simulink model "PID666"  (R2024b)
settings: Solver=FixedStepDiscrete  StartTime=0.0  StopTime=inf  FixedStep=0.0001  RelTol=1e-3
undefined symbols (not defined in the file or in its folder): C28x, CPU1, CPU2, dspblkCoreblockFVToolHelper, gcbh
libraries: c2837xDlib x5, c280xlib x2, c2802xlib x1
settings Model: SimulationMode=external  ExtModeTrigDuration=8  Creator=lenovo  LastModifiedBy=chaiy
settings OptimizationCC: DefaultUnderspecifiedDataType=single  EnhancedBackFolding=on  PassReuseOutputArgsAs=Individual arguments  MaxStackSize=1024  OptimizeBlockOrder=speed  DifferentSizesBufferReuse=on  OptimizationCustomize=off  DenormalBehavior=FlushToZero  EfficientTunableParamExpr=on
settings DebuggingCC: ParameterTunabilityLossMsg=error
settings HardwareCC: ProdBitPerChar=16  ProdBitPerInt=16  ProdBitPerPointer=32  ProdBitPerSizeT=32  ProdBitPerPtrDiffT=32  ProdLargestAtomicInteger=Integer  ProdLargestAtomicFloat=None  ProdWordSize=16  ProdLongLongMode=on  ProdHWDeviceType=Texas Instruments->C2000
settings ModelReferenceCC: EnableRefExpFcnMdlSchedulingChecks=on  ModelReferenceNumInstancesAllowed=Single
settings SFSimCC: MATLABDynamicMemAlloc=off
settings RTWCC: Description=Embedded Coder  SystemTargetFile=ert.tlc  HardwareBoard=TI Delfino F28379D LaunchPad  TemplateMakefile=ert_default_tmf  Toolchain=Texas Instruments Code Composer Studio (C2000)  CodeProfilingSaveOptions=AllData  GPUComputeCapability=3.5
settings CodeAppCC: ForceParamTrailComments=on  IgnoreCustomStorageClasses=off  MaxIdLength=95  OperatorAnnotations=on  SimulinkDataObjDesc=on  SFDataObjDesc=on  InsertBlockDesc=on
settings ERTTargetCC: CodeReplacementLibrary=TI C28x  SupportContinuousTime=on  ExtMode=on  ExtModeTransport=4  ExtModeStaticAlloc=on  ExtModeMexFile=ext_xcp  ExtModeIntrfLevel=Level2 - Open  InlinedParameterPlacement=Hierarchical  DynamicArrayContainerType=coder::array

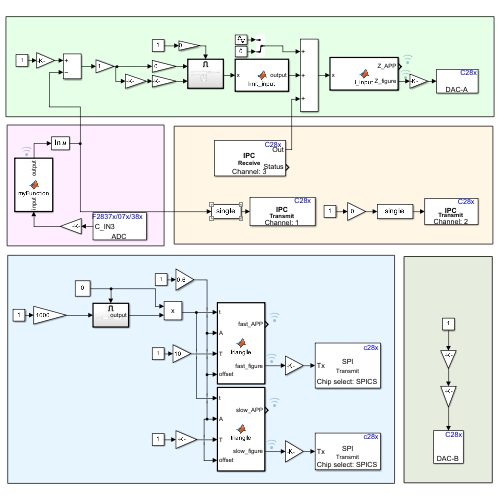
[thumbnail: Simulink's stored preview of the top-level diagram]
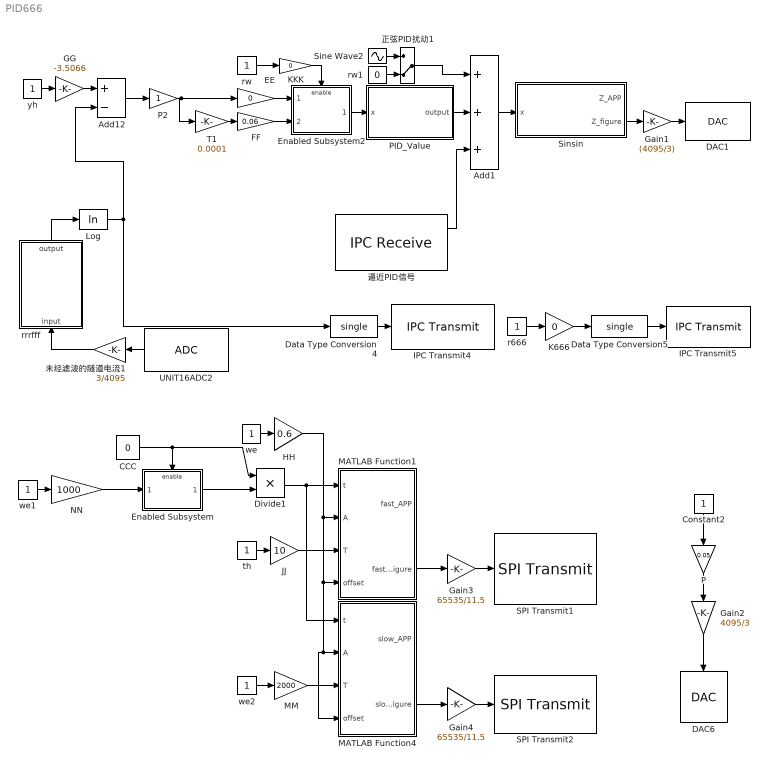
== system PID666 ==
  Add1 : Sum  Inputs=+++
  Add12 : Sum  Inputs=+-
  CCC : Constant  Value=0  SampleTime=0.0001
  Constant2 : Constant  SampleTime=0.0001
  DAC1 : c2837xDlib/DAC  channel=A  saturate=off
  DAC6 : c2837xDlib/DAC  channel=B  saturate=off
  Data Type Conversion4 : DataTypeConversion  OutDataTypeStr=single  SaturateOnIntegerOverflow=off  RndMeth=Floor
  Data Type Conversion5 : DataTypeConversion  OutDataTypeStr=single  SaturateOnIntegerOverflow=off  RndMeth=Floor
  Divide1 : Product  Inputs=**
  EE : Gain  Gain=0
  Enabled Subsystem : Subsystem  TreatAsAtomicUnit=on
  Enabled Subsystem2 : Subsystem  TreatAsAtomicUnit=on
  FF : Gain  Gain=0.06
  GG : Gain  Gain=-3.5066
  Gain1 : Gain  Gain=(4095/3)
  Gain2 : Gain  Gain=4095/3
  Gain3 : Gain  Gain=65535/11.5  OutDataTypeStr=uint16
  Gain4 : Gain  Gain=65535/11.5  OutDataTypeStr=uint16
  HH : Gain  Gain=0.6
  IPC Transmit4 : c2837xDlib/IPC Transmit  blkParamProc=F2837x  SelectDestination=C28x (CPU1/CPU2)  SelectChannel=1  EnableBlocking=off
  IPC Transmit5 : c2837xDlib/IPC Transmit  blkParamProc=F2837x  SelectDestination=C28x (CPU1/CPU2)  SelectChannel=2  EnableBlocking=off
  JJ : Gain  Gain=10
  K666 : Gain  Gain=0
  KKK : Gain  Gain=0
  Log : Math  Operator=log  OutputSignalType=real
  MATLAB Function1 : MATLAB Function  TreatAsAtomicUnit=on
  MATLAB Function4 : MATLAB Function  TreatAsAtomicUnit=on
  MM : Gain  Gain=2000
  NN : Gain  Gain=1000
  P : Gain  Gain=0.05
  P2 : Gain
  PID_Value : MATLAB Function  TreatAsAtomicUnit=on
  SPI Transmit1 : c280xlib/SPI Transmit  SPISelect=SPI_A  ClockPolarity=Rising_edge  ClockPhase=No_delay  SPIModule=uint32(0)  Mode=Master  BusSpeed=uint32(1000000)  FirstBitToTransfer=Most significant bit (MSB)  ClockMode=0  BlockFunction=Write  EnableRegisterAddress=on  RegisterAddress=0  OutputDataType=int8  OutputDataLength=1  BlockingMode=on  DataBits=16  UseCustomSSPin=Provided by the SPI peripheral  ActiveLowSSPin=Active low  Pin=0
  SPI Transmit2 : c280xlib/SPI Transmit  SPISelect=SPI_B  ClockPolarity=Rising_edge  ClockPhase=No_delay  SPIModule=uint32(0)  Mode=Master  BusSpeed=uint32(1000000)  FirstBitToTransfer=Most significant bit (MSB)  ClockMode=0  BlockFunction=Write  EnableRegisterAddress=on  RegisterAddress=0  OutputDataType=int8  OutputDataLength=1  BlockingMode=on  DataBits=16  UseCustomSSPin=Provided by the SPI peripheral  ActiveLowSSPin=Active low  Pin=0
  Sine Wave2 : Sin  SineType=Sample based  Amplitude=0.1  Bias=0.1  Samples=1000  SampleTime=0.0001
  Sinsin : MATLAB Function  TreatAsAtomicUnit=on
  T1 : Gain  Gain=0.0001
  UNIT16ADC2 : c2802xlib/ADC  blkParamProc=C2000_Type4  ADCModule=C  samplingMode=Single sample mode  ADCResolution=12-bit (Single-ended input)  useSOC1=SOC0  useSOC2=SOC0_SOC1  SOCAcquisitionWindow=15  SOCTriggerSource=Software  SOCInterruptTrigger=No ADCINT  Ts=0.0001  dType=double  postInterrupt=off  interruptSel=ADCINT1  ADCINTContinuous=on  endma=off  chdma=1  conv1=ADCINA0  conv2=ADCINA0 and ADCINB0  conv1_Type4=ADCIN3  conv2_Type4=ADCIN0 and ADCIN1
  r666 : Constant  SampleTime=0.0001
  rrrfff : MATLAB Function  TreatAsAtomicUnit=on
  rw : Constant  SampleTime=0.0001
  rw1 : Constant  Value=0  SampleTime=0.0001
  th : Constant  SampleTime=0.0001
  we : Constant  SampleTime=0.0001
  we1 : Constant  SampleTime=0.0001
  we2 : Constant  SampleTime=0.0001
  yh : Constant  SampleTime=0.0001
  未经滤波的隧道电流1 : Gain  Gain=3/4095
  正弦PID扰动1 : ManualSwitch  CurrentSetting=0
  逼近PID信号 : c2837xDlib/IPC Receive  blkParamProc=F2837x  SelectSource=C28x (CPU1/CPU2)  SelectChannel=3  DataType=single  DataLength=1  EnableBlocking=off  SampleTime=0.0001
  wires:
  Divide1/1 -> MATLAB Function4/1(t), MATLAB Function1/1(t)
  JJ/1 -> MATLAB Function1/3(T)
  Enabled Subsystem/1(output) -> Divide1/2
  HH/1 -> MATLAB Function4/4(offset), MATLAB Function4/2(A), MATLAB Function1/4(offset), MATLAB Function1/2(A)
  Constant2/1 -> P/1
  we/1 -> HH/1
  th/1 -> JJ/1
  MM/1 -> MATLAB Function4/3(T)
  GG/1 -> Add12/1
  T1/1 -> FF/1
  rrrfff/1(output) -> Log/1
  EE/1 -> Enabled Subsystem2/1(比例模块)
  KKK/1 -> Enabled Subsystem2/Enable
  FF/1 -> Enabled Subsystem2/2(积分模块)
  P2/1 -> T1/1, EE/1
  UNIT16ADC2/1 -> 未经滤波的隧道电流1/1
  Enabled Subsystem2/1(output) -> PID_Value/1(x)
  Add12/1 -> P2/1
  yh/1 -> GG/1
  rw/1 -> KKK/1
  CCC/1 -> Enabled Subsystem/Enable, Divide1/1
  Gain3/1 -> SPI Transmit1/1
  Gain4/1 -> SPI Transmit2/1
  Gain1/1 -> DAC1/1
  P/1 -> Gain2/1
  Gain2/1 -> DAC6/1
  we1/1 -> NN/1
  we2/1 -> MM/1
  NN/1 -> Enabled Subsystem/1(持续时间(s))
  Sinsin/2(Z_figure) -> Gain1/1
  Add1/1 -> Sinsin/1(x)
  PID_Value/1(output) -> Add1/2
  Sine Wave2/1 -> 正弦PID扰动1/1
  rw1/1 -> 正弦PID扰动1/2
  正弦PID扰动1/1 -> Add1/1
  Data Type Conversion5/1 -> IPC Transmit5/1
  Log/1 -> Data Type Conversion4/1, Add12/2
  逼近PID信号/1 -> Add1/3
  K666/1 -> Data Type Conversion5/1
  Data Type Conversion4/1 -> IPC Transmit4/1
  r666/1 -> K666/1
  MATLAB Function1/2(fast_figure) -> Gain3/1
  MATLAB Function4/2(slow_figure) -> Gain4/1
  未经滤波的隧道电流1/1 -> rrrfff/1(input)

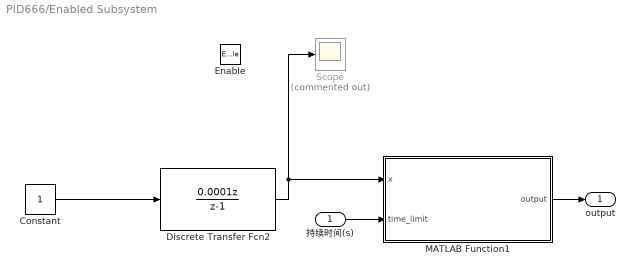
== system PID666/Enabled Subsystem ==
  持续时间(s) : Inport
  Enable : EnablePort  StatesWhenEnabling=reset
  Constant : Constant  SampleTime=1/10000
  Discrete Transfer Fcn2 : DiscreteTransferFcn  LoadFcn=dspblkCoreblockFVToolHelper(gcbh,'load');  Numerator=[0.0001 0]  Denominator=[1 -1]  SampleTime=0.0001
      settings: CopyFcn=dspblkCoreblockFVToolHelper(gcbh,'copy');  DeleteFcn=dspblkCoreblockFVToolHelper(gcbh,'close');  ModelCloseFcn=dspblkCoreblockFVToolHelper(gcbh,'close');  PreSaveFcn=dspblkCoreblockFVToolHelper(gcbh,'presave');  PostSaveFcn=dspblkCoreblockFVToolHelper(gcbh,'postsave');  CloseFcn=dspblkCoreblockFVToolHelper(gcbh,'close');
  MATLAB Function1 : MATLAB Function  TreatAsAtomicUnit=on
  Scope : Scope  Commented=on
  output : Outport
  wires:
  Constant/1 -> Discrete Transfer Fcn2/1
  Discrete Transfer Fcn2/1 -> Scope/1, MATLAB Function1/1(x)
  持续时间(s)/1 -> MATLAB Function1/2(time_limit)
  MATLAB Function1/1(output) -> output/1

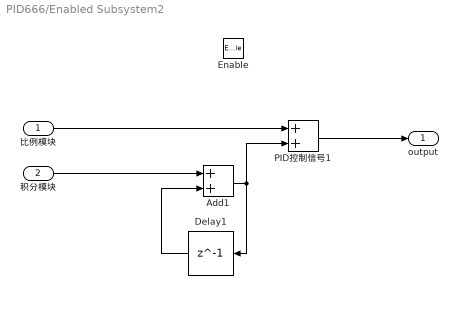
== system PID666/Enabled Subsystem2 ==
  比例模块 : Inport
  积分模块 : Inport  Port=2
  Enable : EnablePort  StatesWhenEnabling=reset
  Add1 : Sum
  Delay1 : Delay  DelayLength=1  SampleTime=0.0001
  PID控制信号1 : Sum
  output : Outport  OutputWhenDisabled=reset  InitialOutput=[0]
  wires:
  PID控制信号1/1 -> output/1
  Add1/1 -> Delay1/1, PID控制信号1/2
  Delay1/1 -> Add1/2
  积分模块/1 -> Add1/1
  比例模块/1 -> PID控制信号1/1

== matlab function PID666/Sinsin ==
  data: x input; Z_APP output; Z_figure output
function [Z_APP,Z_figure] = l_input(x)

    Z_APP = x;
    Z_figure = x;

end

== matlab function PID666/MATLAB Function4 ==
  data: t input; slow_APP output; A input; T input; offset input; slow_figure output
function [slow_APP,slow_figure ] = triangle(t,A,T,offset)
% triangle - 产生幅值 A、频率 f、相位 phi 的三角波
%  输入: t —— 当前仿真时间（从 Clock 块接入）
%  输出: y —— 三角波值

% A = 1;        % 幅值
% f = 10;        % 频率 (Hz)
% phi = 0;      % 相位 (rad)
degrees = 270;
phi = degrees * (pi / 180);


f = 1/T;

% 用 asin(sin(...)) 公式生成标准三角波，区间 [-A, A]
y = A * (2/pi) * asin( sin( 2*pi*f*t + phi ) );

y = y + offset;


slow_figure = y;
slow_APP = y;

== matlab function PID666/Enabled Subsystem/MATLAB Function1 ==
  data: x input; output output; time_limit input
function output = limit_min_zero(x,time_limit)

    output = min(x, time_limit);

end

== matlab function PID666/PID_Value ==
  data: x input; output output
function output = limit_input(x)

    output = min(x, 3);

end

== matlab function PID666/rrrfff ==
  data: input input; output output

function output = myFunction(input)
    if input == 0
        output = 0.002;
    else
        output = input;
    end
end

== matlab function PID666/MATLAB Function1 ==
  data: t input; fast_APP output; A input; T input; offset input; fast_figure output
function [fast_APP,fast_figure ]= triangle(t,A,T,offset)
% triangle - 产生幅值 A、频率 f、相位 phi 的三角波
%  输入: t —— 当前仿真时间（从 Clock 块接入）
%  输出: y —— 三角波值

% A = 1;        % 幅值
% f = 10;        % 频率 (Hz)
% phi = 0;      % 相位 (rad)
degrees = 270;
phi = degrees * (pi / 180);


f = 1/T;

% 用 asin(sin(...)) 公式生成标准三角波，区间 [-A, A]
y = A * (2/pi) * asin( sin( 2*pi*f*t + phi ) );

y = y + offset;



fast_APP = y;
fast_figure = y;
